simulink model "homework_2_simulation_simulink"  (R2018b)
settings: Solver=ode1  StartTime=0.0  StopTime=100  FixedStep=0.009  RelTol=1e-3
settings Model: Creator=Eduardo  LastModifiedBy=Eduardo

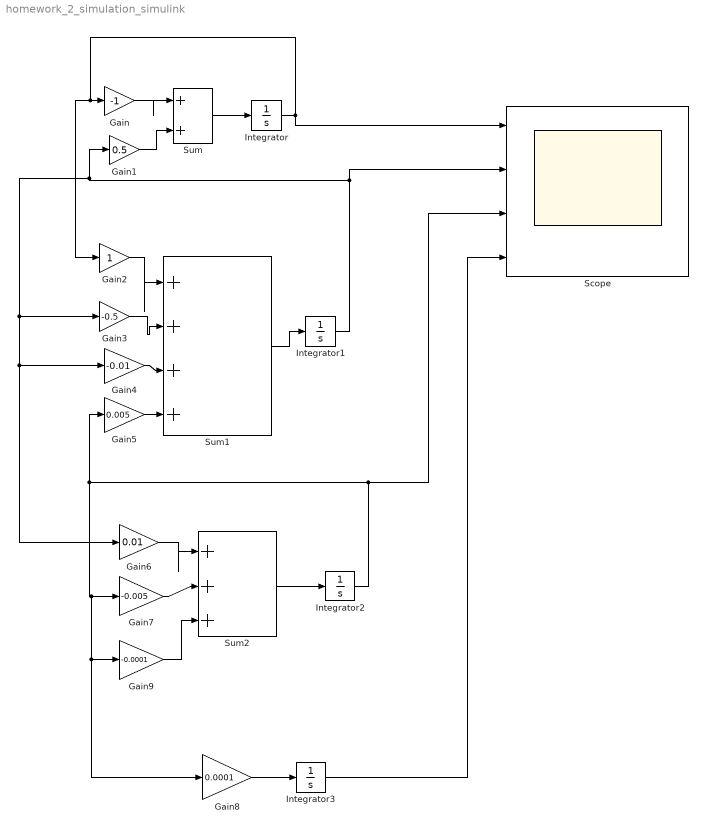
== system homework_2_simulation_simulink ==
  Gain : Gain  Gain=-1
  Gain1 : Gain  Gain=0.5
  Gain2 : Gain
  Gain3 : Gain  Gain=-0.5
  Gain4 : Gain  Gain=-0.01
  Gain5 : Gain  Gain=0.005
  Gain6 : Gain  Gain=0.01
  Gain7 : Gain  Gain=-0.005
  Gain8 : Gain  Gain=0.0001
  Gain9 : Gain  Gain=-0.0001
  Integrator : Integrator  InitialCondition=1
  Integrator1 : Integrator
  Integrator2 : Integrator
  Integrator3 : Integrator
  Scope : Scope  NumInputPorts=4
  Sum : Sum  Inputs=|++
  Sum1 : Sum  Inputs=|++++
  Sum2 : Sum  Inputs=|+++
  wires:
  Gain/1 -> Sum/1
  Gain1/1 -> Sum/2
  Sum/1 -> Integrator/1
  Integrator/1 -> Gain2/1, Gain/1, Scope/1
  Sum1/1 -> Integrator1/1
  Gain2/1 -> Sum1/1
  Gain3/1 -> Sum1/2
  Integrator1/1 -> Scope/2, Gain6/1, Gain4/1, Gain3/1, Gain1/1
  Gain4/1 -> Sum1/3
  Gain5/1 -> Sum1/4
  Sum2/1 -> Integrator2/1
  Gain6/1 -> Sum2/1
  Gain7/1 -> Sum2/2
  Integrator2/1 -> Gain5/1, Gain8/1, Gain9/1, Gain7/1, Scope/3
  Gain9/1 -> Sum2/3
  Gain8/1 -> Integrator3/1
  Integrator3/1 -> Scope/4
